simulink model "Lead_Acid_Battery"  (R2024b)
settings: Solver=ode23  StartTime=0.0  StopTime=5  RelTol=1e-3
settings Model: Creator=10537  LastModifiedBy=10537

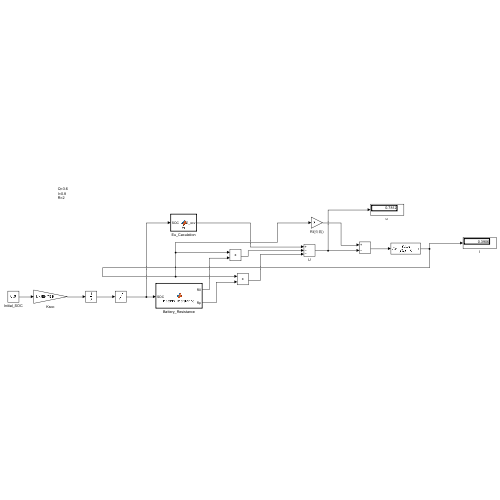
[thumbnail: Simulink's stored preview of the top-level diagram]
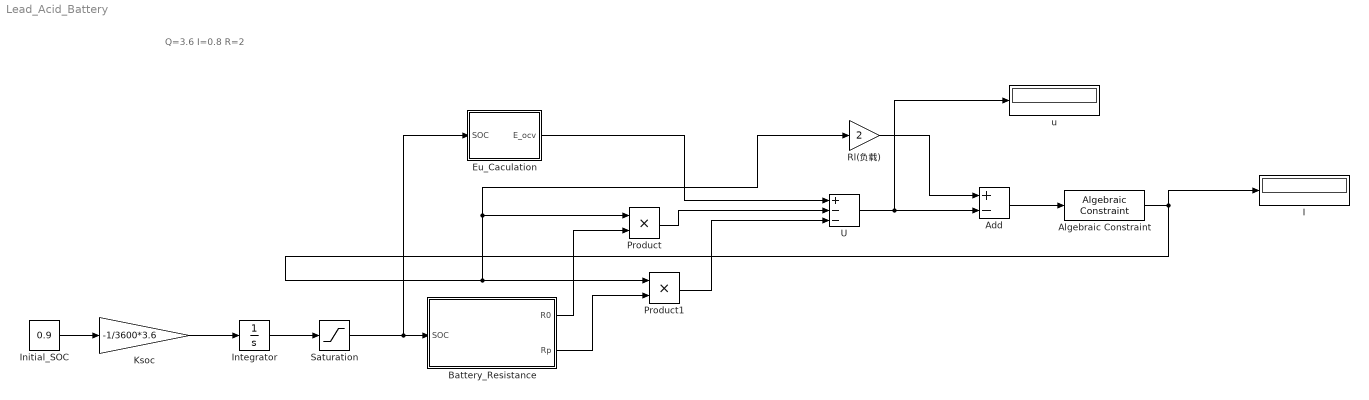
== system Lead_Acid_Battery ==
  note: Q=3.6
      | I=0.8
      | R=2
  Add : Sum  Inputs=+-
  Algebraic Constraint : AlgebraicConstraint  InitialGuess=0.8
  Battery_Resistance : MATLAB Function  TreatAsAtomicUnit=on
  Eu_Caculation : MATLAB Function  TreatAsAtomicUnit=on
  I : Display
  Initial_SOC : Constant  Value=0.9
  Integrator : Integrator
  Ksoc : Gain  Gain=-1/3600*3.6
  Product : Product
  Product1 : Product
  Rl(负载) : Gain  Gain=2
  Saturation : Saturate  UpperLimit=1  LowerLimit=0
  U : Sum  Inputs=+--
  "u " : Display
  wires:
  Battery_Resistance/1(R0) -> Product/2
  Battery_Resistance/2(Rp) -> Product1/2
  Product/1 -> U/2
  Product1/1 -> U/3
  U/1 -> "u "/1, Add/2
  Algebraic Constraint/1 -> Product1/1, Rl(负载)/1, Product/1, I/1
  Saturation/1 -> Eu_Caculation/1(SOC), Battery_Resistance/1(SOC)
  Eu_Caculation/1(E_ocv) -> U/1
  Rl(负载)/1 -> Add/1
  Add/1 -> Algebraic Constraint/1
  Ksoc/1 -> Integrator/1
  Integrator/1 -> Saturation/1
  Initial_SOC/1 -> Ksoc/1

== matlab function Lead_Acid_Battery/Battery_Resistance ==
  data: SOC input; R0 output; Rp output
function [R0, Rp] = battery_resistance(SOC)
    % 电池的欧姆内阻 R0（根据二次曲线拟合）
    a0 = 0.5; a1 = 0.1; a2 = -0.02;  
    R0 = a0 + a1 * SOC + a2 * SOC^2;

    % 电池的极化内阻 Rp（根据指数曲线拟合）
    b0 = 0.05; b1 = 3; b2 = 0.01;  
    Rp = b0 * exp(-b1 * SOC) + b2;
end

== matlab function Lead_Acid_Battery/Eu_Caculation ==
  data: SOC input; E_ocv output
function E_ocv = f1(SOC)
    % 电池的开路电压E_ocv与SOC的多项式关系
    E_ocv = 3.7 * SOC^3 - 0.8 * SOC^2 + 2.1 * SOC + 1.0;  % 拟合多项式
end
